simulink model "trippel_oppdatert_sim"  (R2023b)
settings: Solver=VariableStepAuto  StartTime=0.0  StopTime=inf  FixedStep=0.0001  RelTol=1e-6  AbsTol=1e-6
model workspace (MAT data in the model file):
  SL_ROS_VariableLengthArrays_MaxSizes.CommonInfo.ArrayTruncateAction = 'EmitWarning'
  SL_ROS_VariableLengthArrays_MaxSizes.MsgTypeMap = containers.Map
  SL_ROS_VariableLengthArrays_MaxSizes.MsgTypeMap.serialization.keys = {'std_msgs/Float64MultiArray'}
  SL_ROS_VariableLengthArrays_MaxSizes.MsgTypeMap.serialization.values{1}.PropertyName = 'data'
  SL_ROS_VariableLengthArrays_MaxSizes.MsgTypeMap.serialization.values{1}.DataType = 'double'
  SL_ROS_VariableLengthArrays_MaxSizes.MsgTypeMap.serialization.values{1}.MaxLength = 500
  SL_ROS_VariableLengthArrays_MaxSizes.MsgTypeMap.serialization.uniformity = 0
  SL_ROS_VariableLengthArrays_MaxSizes.MsgTypeMap.serialization.keyType = 'char'
  SL_ROS_VariableLengthArrays_MaxSizes.MsgTypeMap.serialization.valueType = 'any'
values from neighbouring files (symbols this model uses):
  Iz = (1/12) * m * (with^2 + len^2)    [LoneWolfParams.m]
  m = 375    [LoneWolfParams.m]
  wheelRadius = 0.33    [LoneWolfParams.m]
  xdotinit = 1e-3    (= 0.001)    [LoneWolfParams.m]
undefined symbols (not defined in the file or in its folder): alpha_peak, Bc, Bl, Cc, Cl, Dc, Dl, Ec, El, kappa_peak, latitude, longitude
libraries: ros2lib x11, sldrtlib x1
settings Model: Creator=bakke  LastModifiedBy=lonewolf
settings SolverCC: AutoScaleAbsTol=off  EnableFixedStepZeroCrossing=on  MaxZcBracketingIterations=100
settings OptimizationCC: EnhancedBackFolding=on  PassReuseOutputArgsAs=Individual arguments  ZeroExternalMemoryAtStartup=off  ZeroInternalMemoryAtStartup=off  MaxStackSize=64  OptimizeBlockOrder=speed  DifferentSizesBufferReuse=on  EfficientTunableParamExpr=on
settings DebuggingCC: ParameterTunabilityLossMsg=error
settings HardwareCC: ProdBitPerLong=64  ProdHWDeviceType=Intel->x86-64 (Linux 64)  UseEmbeddedCoderFeatures=off
settings RTWCC: Description=Embedded Coder  SystemTargetFile=ert.tlc  HardwareBoard=Robot Operating System 2 (ROS 2)  TLCOptions="-aInlineSetEventsForThisBaseRateFcn=TLC_FALSE -aSuppressMultiTaskScheduler=TLC_FALSE  -aRateBasedStepFcn=0"  TemplateMakefile=ert_default_tmf  Toolchain=Colcon Tools  TargetLang=C++
settings CodeAppCC: ForceParamTrailComments=on  IgnoreCustomStorageClasses=off  OperatorAnnotations=on  SimulinkDataObjDesc=on  SFDataObjDesc=on  InsertBlockDesc=on
settings ERTTargetCC: CodeInterfacePackaging=C++ class  SupportNonInlinedSFcns=on  RootIOFormat=Structure reference

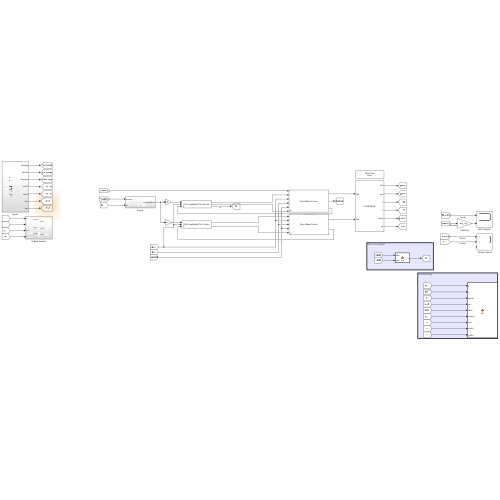
[thumbnail: Simulink's stored preview of the top-level diagram]
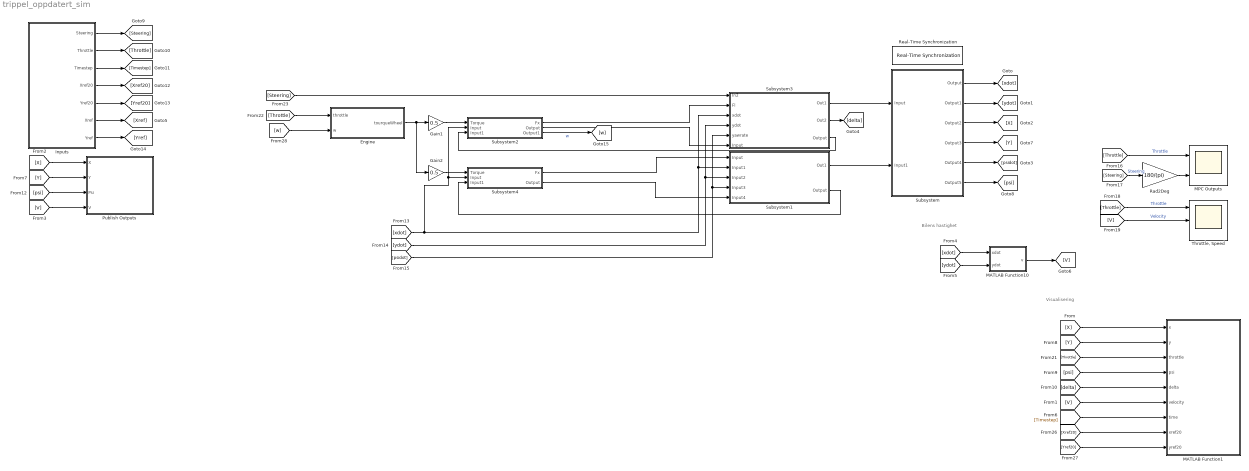
== system trippel_oppdatert_sim ==
  note: Visualisering
  note: Bilens hastighet
  Engine : Subsystem
  Gain1 : Gain  Gain=0.5
  Gain2 : Gain  Gain=0.5
  Inputs : Subsystem
  MATLAB Function1 : MATLAB Function  TreatAsAtomicUnit=on
  MATLAB Function10 : MATLAB Function  TreatAsAtomicUnit=on
  MPC Outputs : Scope  NumInputPorts=2
  Publish Outputs : Subsystem
  Rad2Deg : Gain  Gain=180/(pi)
  Real-Time Synchronization : sldrtlib/Real-Time Synchronization  SampleTime=0.1  MaxMissedTicks=1000  ShowMissedTicks=off  YieldWhenWaiting=off
  Subsystem : Subsystem
      mask Display: disp('LONE WOLF');
  Subsystem1 : Subsystem
      mask Display: disp('Rear Wheel Forces');
  Subsystem2 : Subsystem
      mask Display: disp('FW Longitudinal Tire Forces');
  Subsystem3 : Subsystem
      mask Display: disp('Front Wheel Forces');
  Subsystem4 : Subsystem
      mask Display: disp('RW Longitudinal Tire Forces');
  "Throttle, Speed" : Scope  NumInputPorts=3
  wires:
  MATLAB Function10/1(v) -> [V]
  [ydot] -> MATLAB Function10/2(ydot)
  Subsystem/1(Output) -> [xdot]
  [xdot] -> MATLAB Function10/1(xdot)
  Subsystem/2(Output1) -> [ydot]
  Subsystem/5(Output4) -> [psidot]
  Subsystem/4(Output3) -> [Y]
  Subsystem/3(Output2) -> [X]
  Subsystem/6(Output5) -> [psi]
  Subsystem1/1(Out1) -> Subsystem/2(Input1)
  Subsystem3/1(Out1) -> Subsystem/1(Input)
  [xdot] -> Subsystem4/2(Input), Subsystem2/2(Input), Subsystem3/3(xdot), Subsystem1/2(Input1)
  [ydot] -> Subsystem1/3(Input2), Subsystem3/4(ydot)
  [psidot] -> Subsystem3/5(yawrate), Subsystem1/4(Input3)
  Subsystem3/2(Out2) -> [delta]
  [X] -> MATLAB Function1/1(x)
  [Y] -> MATLAB Function1/2(y)
  [psi] -> MATLAB Function1/4(psi)
  [delta] -> MATLAB Function1/5(delta)
  [X] -> Publish Outputs/1(X)
  [Y] -> Publish Outputs/2(Y)
  [psi] -> Publish Outputs/3(Psi)
  [V] -> Publish Outputs/4(V)
  [V] -> MATLAB Function1/6(velocity)
  Inputs/1(Steering) -> [Steering]
  Inputs/2(Throttle) -> [Throttle]
  [Throttle] -> MPC Outputs/1  "Throttle"
  [Steering] -> Rad2Deg/1  "Steering"
  [Throttle] -> "Throttle, Speed"/1  "Throttle"
  [V] -> "Throttle, Speed"/2  "Velocity"
  Rad2Deg/1 -> MPC Outputs/2
  Inputs/3(Timestep) -> [Timestep]
  Inputs/4(Xref20) -> [Xref20]
  Inputs/5(Yref20) -> [Yref20]
  Subsystem2/1(Fx) -> Subsystem3/2(Fl)
  Gain1/1 -> Subsystem2/1(Torque)
  Engine/1(tourqueWheel) -> Gain2/1, Gain1/1
  Gain2/1 -> Subsystem4/1(Torque)
  Subsystem2/2(Output) -> Subsystem3/6(Input)
  Subsystem4/1(Fx) -> Subsystem1/1(Input)
  Subsystem4/2(Output) -> Subsystem1/5(Input4)
  Inputs/6(Xref) -> [Xref]
  Inputs/7(Yref) -> [Yref]
  Subsystem2/3(Output1) -> [w]  "w"
  [Steering] -> Subsystem3/1(In2)
  [w] -> Engine/2(w)
  Subsystem1/2(Output) -> Subsystem4/3(Input1)
  Subsystem3/3(Output) -> Subsystem2/3(Input1)
  [Yref20] -> MATLAB Function1/9(yref20)
  [Xref20] -> MATLAB Function1/8(xref20)
  [Throttle] -> MATLAB Function1/3(throttle)
  [Timestep] -> MATLAB Function1/7(time)
  [Throttle] -> Engine/1(throttle)

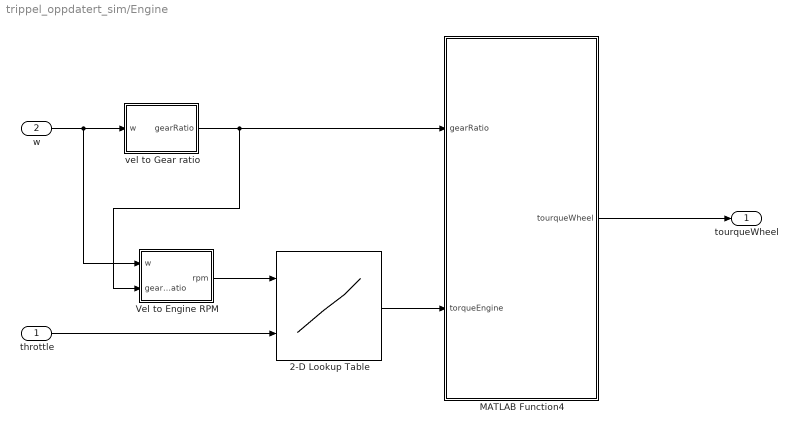
== system trippel_oppdatert_sim/Engine ==
  throttle : Inport
  w : Inport  Port=2
  2-D Lookup Table : Lookup_n-D  BreakpointsForDimension1=[0;169.614855264094;367.085957899886;589.246670617181;789.821522752712;996.567251474744;1181.71186027627;1425.48895225281;1626.06685625609;1835.92854194885;2042.68342627413;2243.26743401291;2425.36017506641;2616.68481605769;2860.48021924071;3085.77825200297;3264.76724355674;3468.45194892751;3656.70641096427;3909.77338836579;4131.97377536381;4314.05736081407;4493.04635236784;4696.71885026762;4909.65376678264;5110.24998199241;5292.32135997168;5499.07014056146;5718.17288179523;5965.03541206502;6199.56534476505;6390.87472641759;6582.16884873138;6758.05409078541;6980.20259603171]  BreakpointsForDimension2=[0;10;20;30;40;50;60;70;80;90;100]  Table=[0.3 7.52683562951347 11.8387627553835 13.7538912505429 14.2370681748395 17.110514311951 18.5474885119643 17.5896731329271 18.0683296909882 19.0271495958556 24.298398889508;0.2 10.3686392029757 12.7749808290727 17.5615464096832 19.4852133743988 21.8820120051095 25.2300965969615 24.7539513534759 28.0985201049223 31.4546409034155 33.8484259566359;0 11.2978255958539 15.1431504736246 22.3255101591157 25.2084992916136 29.038254019017 37.6505562237105 34.7881598707304 46.2688855833847 47.2272032253369 51.5386280882919;0 13.1858318935994 20.8624182875188 30.4380607633152 37.1492978344714 39.5491100426724 54.8631063231358 53.915838465315 65.4061071733557 67.8013990153211 73.0706392573133;0 16.0346671478725 30.4094317771563 43.3462176805965 52.4527465937181 63.4723949503387 69.6994505713682 77.3680007586463 84.553876284543 88.8678124620733 88.8688169879034;-2.44629412790408 24.6344127796893 47.1563841543122 73.0294536982776 73.0379921678338 91.720665819667 102.743327753778 118.552053005585 116.160277004025 127.660088707451 124.308990538109;-4.96800884998436 35.1502914324955 71.0816781136389 103.177785175313 114.222546677687 132.430079611865 148.722986313798 180.336920977006 188.48362545943 193.279734035427 163.107293938468;-8.74578514092923 33.6856927721534 72.4880142758329 104.587637177913 130.961462848202 155.87470796147 177.437859431226 195.635347107102 209.529446126664 221.029760093006 226.319090851601;-12.1015317204333 33.6520411568438 75.3288133234649 113.858360154898 143.370370427905 164.462399283325 190.810609544946 214.287382721116 229.13779033097 243.993220569975 247.83502960734;-19.201920026761 35.0558660044625 81.0551128181702 121.980453754484 158.198176206581 185.034586021649 211.865973207567 232.947956804686 250.676330917887 265.053104598831 277.032075123234;-23.3903905203684 35.0282415441337 84.3810978417591 127.227594428213 165.359943112554 196.510289105152 225.735461344291 249.691393341436 267.899930801444 284.190326188802 296.649460060012;-27.5779890517621 31.4144554912304 86.2680996136746 133.424012011423 173.479023134649 206.067347853091 234.811352219593 263.073686450543 283.200365983201 296.143179041622 314.343680294988;-34.6744535281279 28.5083622646395 84.8029986904173 132.424508810435 174.403689161292 210.348636941142 239.083600575173 265.9119741836 288.438465924458 303.782095716911 318.144303773318;-38.4448181402563 22.7303296896822 79.0219525379695 127.60881198075 170.065644363838 207.922707061357 236.655159380812 261.571418071571 285.059241031872 302.791633248394 315.243735438792;-44.7181502868699 19.3501002712657 76.5965249210998 125.188909255946 170.034504063104 205.489745500762 237.114227685186 262.989306280812 284.552457750567 303.239651768636 317.613914135005;-53.0684964265662 14.5328966528359 72.7336208413018 123.725817384349 168.093257896361 204.501292083905 235.646615447353 263.444356481864 285.961807490252 304.168335898599 318.061932655246;-57.6689690661566 10.1943495924673 67.9169194857871 119.863917830381 165.197712190987 201.122569454234 232.254331718975 261.012399447099 284.010516065207 301.740396967154 318.513467015894;-63.9366334583809 4.41481022876471 62.1353710704242 114.762859997277 162.775298151607 195.485378400082 228.870586460153 255.707498538137 277.747799777208 296.440518687343 312.256777882875;-69.7861919691262 -2.32304677689018 58.7496167599421 109.939629223867 157.474917608881 193.058946257382 225.968009073968 255.203226571407 278.19581829745 296.410885175354 312.707307717692;-78.1404619387842 -9.54508523267177 53.452249794706 105.592543693942 154.556770072328 190.157373397027 224.031785536375 252.782821583688 275.782444990542 295.429463439308 311.718854300836;-84.8266681935945 -12.4471603559423 48.6390642795968 102.692979885247 151.179554231402 188.687752107534 223.0493592745 251.318725186261 274.317344067285 293.481687854669 309.292422158136;-90.6753547421262 -16.3085576469951 45.7379936821564 99.7888957103159 147.799324812986 188.655607280969 222.54508730777 250.807923801635 ...(+2434 chars)]  InternalRulePriority=Speed  RndMeth=Simplest
      settings: InputPortMap=u0,u1
  MATLAB Function4 : MATLAB Function  TreatAsAtomicUnit=on
  Vel to Engine RPM : MATLAB Function  TreatAsAtomicUnit=on
  vel to Gear ratio : MATLAB Function  TreatAsAtomicUnit=on
  tourqueWheel : Outport
  wires:
  vel to Gear ratio/1(gearRatio) -> Vel to Engine RPM/2(gearRatio), MATLAB Function4/1(gearRatio)
  2-D Lookup Table/1 -> MATLAB Function4/2(torqueEngine)
  MATLAB Function4/1(tourqueWheel) -> tourqueWheel/1
  throttle/1 -> 2-D Lookup Table/2
  w/1 -> vel to Gear ratio/1(w), Vel to Engine RPM/1(w)
  Vel to Engine RPM/1(rpm) -> 2-D Lookup Table/1

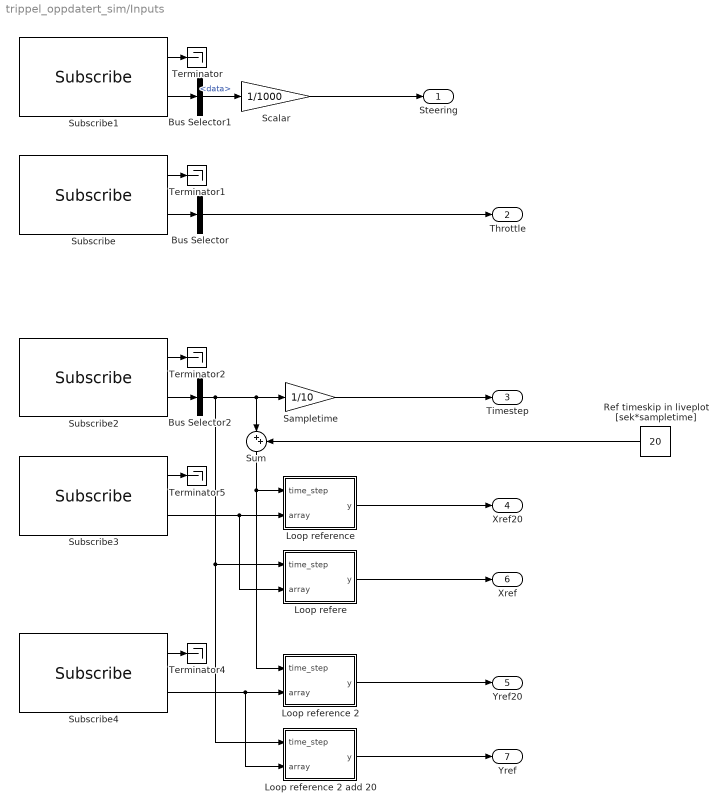
== system trippel_oppdatert_sim/Inputs ==
  Bus Selector : BusSelector  OutputSignals=data  OutputAsBus=on
  Bus Selector1 : BusSelector  OutputSignals=data
  Bus Selector2 : BusSelector  OutputSignals=data  OutputAsBus=on
  Loop refere : MATLAB Function  TreatAsAtomicUnit=on
  Loop reference : MATLAB Function  TreatAsAtomicUnit=on
  Loop reference 2 : MATLAB Function  TreatAsAtomicUnit=on
  Loop reference 2 add 20 : MATLAB Function  TreatAsAtomicUnit=on
  Ref timeskip in liveplot [sek*sampletime] : Constant  Value=20
  Sampletime : Gain  Gain=1/10
  Scalar : Gain  Gain=1/1000
  Subscribe : ros2lib/Subscribe  topicSource=Specify your own  topic=/lw_portenta_throttle  messageType=std_msgs/Int64  sampleTime=0.1  QOSHistory=Keep last  QOSDepth=1  QOSReliability=Reliable  QOSDurability=Volatile
  Subscribe1 : ros2lib/Subscribe  topicSource=Specify your own  topic=/lw_portenta_steering  messageType=std_msgs/Int64  sampleTime=0.1  QOSHistory=Keep last  QOSDepth=1  QOSReliability=Reliable  QOSDurability=Volatile
  Subscribe2 : ros2lib/Subscribe  topicSource=Specify your own  topic=/timestep  messageType=std_msgs/Int64  sampleTime=0.1  QOSHistory=Keep last  QOSDepth=1  QOSReliability=Reliable  QOSDurability=Volatile
  Subscribe3 : ros2lib/Subscribe  topicSource=Specify your own  topic=/xref  messageType=std_msgs/Float64MultiArray  sampleTime=0.1  QOSHistory=Keep last  QOSDepth=1  QOSReliability=Reliable  QOSDurability=Volatile
  Subscribe4 : ros2lib/Subscribe  topicSource=Specify your own  topic=/yref  messageType=std_msgs/Float64MultiArray  sampleTime=0.1  QOSHistory=Keep last  QOSDepth=1  QOSReliability=Reliable  QOSDurability=Volatile
  Sum : Sum  Inputs=|++
  Terminator{,1..2,4..5} (5 alike) : Terminator
  Steering : Outport
  Throttle : Outport  Port=2
  Timestep : Outport  Port=3
  Xref20 : Outport  Port=4
  Yref20 : Outport  Port=5
  Xref : Outport  Port=6
  Yref : Outport  Port=7
  wires:
  Subscribe/1 -> Terminator1/1
  Subscribe1/1 -> Terminator/1
  Subscribe/2 -> Bus Selector/1
  Subscribe1/2 -> Bus Selector1/1
  Bus Selector1/1 -> Scalar/1  "<data>"
  Bus Selector/1 -> Throttle/1
  Scalar/1 -> Steering/1
  Subscribe2/1 -> Terminator2/1
  Subscribe2/2 -> Bus Selector2/1
  Bus Selector2/1 -> Loop refere/1(time_step), Loop reference 2 add 20/1(time_step), Sum/1, Sampletime/1
  Sampletime/1 -> Timestep/1
  Subscribe4/1 -> Terminator4/1
  Subscribe4/2 -> Loop reference 2 add 20/2(array), Loop reference 2/2(array)
  Subscribe3/2 -> Loop refere/2(array), Loop reference/2(array)
  Subscribe3/1 -> Terminator5/1
  Ref timeskip in liveplot [sek*sampletime]/1 -> Sum/2
  Sum/1 -> Loop reference/1(time_step), Loop reference 2/1(time_step)
  Loop reference/1(y) -> Xref20/1
  Loop refere/1(y) -> Xref/1
  Loop reference 2 add 20/1(y) -> Yref/1
  Loop reference 2/1(y) -> Yref20/1

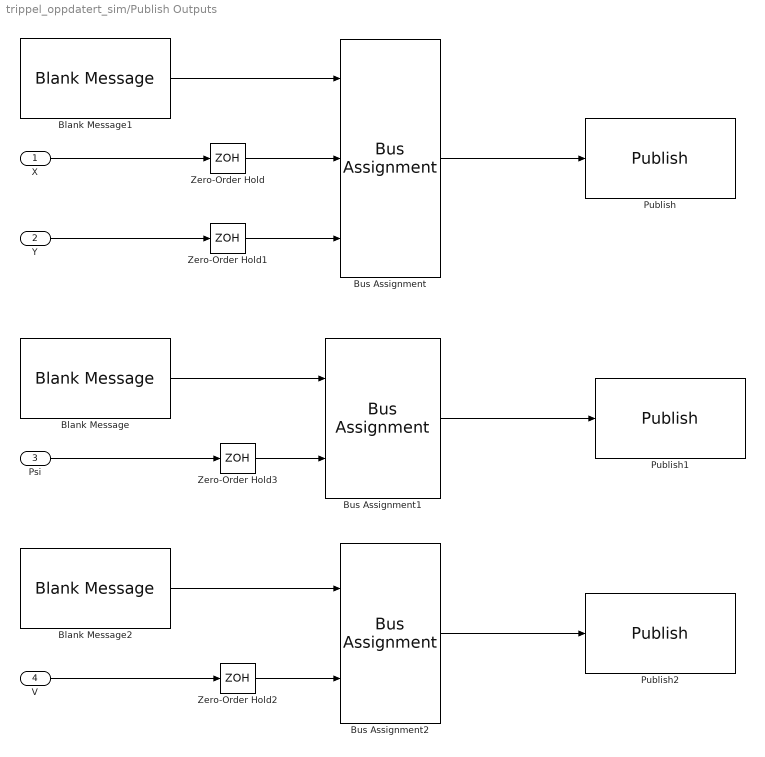
== system trippel_oppdatert_sim/Publish Outputs ==
  X : Inport
  Y : Inport  Port=2
  Psi : Inport  Port=3
  V : Inport  Port=4
  Blank Message : ros2lib/Blank Message  messageClass=Message  entityType=geometry_msgs/PoseWithCovarianceStamped  messageType=geometry_msgs/PoseWithCovarianceStamped  SampleTime=0.1
  Blank Message1 : ros2lib/Blank Message  messageClass=Message  entityType=sensor_msgs/NavSatFix  messageType=sensor_msgs/NavSatFix  SampleTime=0.1
  Blank Message2 : ros2lib/Blank Message  messageClass=Message  entityType=geometry_msgs/TwistWithCovarianceStamped  messageType=geometry_msgs/TwistWithCovarianceStamped  SampleTime=0.1
  Bus Assignment : BusAssignment  AssignedSignals=latitude,longitude
  Bus Assignment1 : BusAssignment  AssignedSignals=pose.pose.position.z
  Bus Assignment2 : BusAssignment  AssignedSignals=twist.twist.linear.x
  Publish : ros2lib/Publish  topicSource=Specify your own  topic=/vectornav/gnss  messageType=sensor_msgs/NavSatFix  QOSHistory=Keep last  QOSDepth=1  QOSReliability=Reliable  QOSDurability=Volatile
  Publish1 : ros2lib/Publish  topicSource=Specify your own  topic=/vectornav/pose  messageType=geometry_msgs/PoseWithCovarianceStamped  QOSHistory=Keep last  QOSDepth=1  QOSReliability=Reliable  QOSDurability=Volatile
  Publish2 : ros2lib/Publish  topicSource=Specify your own  topic=/vectornav/velocity_body  messageType=geometry_msgs/TwistWithCovarianceStamped  QOSHistory=Keep last  QOSDepth=1  QOSReliability=Reliable  QOSDurability=Volatile
  Zero-Order Hold{,1..3} (4 alike) : ZeroOrderHold  SampleTime=0.1
  wires:
  Blank Message/1 -> Bus Assignment1/1
  Bus Assignment1/1 -> Publish1/1
  Zero-Order Hold2/1 -> Bus Assignment2/2
  Bus Assignment2/1 -> Publish2/1
  Zero-Order Hold3/1 -> Bus Assignment1/2
  Psi/1 -> Zero-Order Hold3/1
  Blank Message1/1 -> Bus Assignment/1
  V/1 -> Zero-Order Hold2/1
  X/1 -> Zero-Order Hold/1
  Zero-Order Hold/1 -> Bus Assignment/2
  Bus Assignment/1 -> Publish/1
  Blank Message2/1 -> Bus Assignment2/1
  Y/1 -> Zero-Order Hold1/1
  Zero-Order Hold1/1 -> Bus Assignment/3

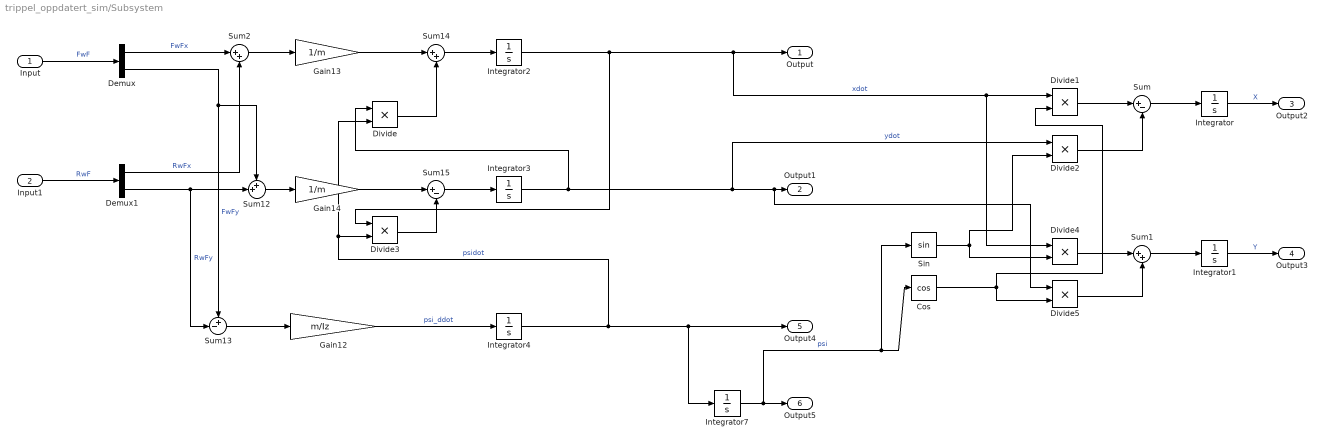
== system trippel_oppdatert_sim/Subsystem ==
  Input : Inport
  Input1 : Inport  Port=2
  Cos : Trigonometry  Operator=cos
  Demux : Demux  Outputs=2
  Demux1 : Demux  Outputs=2
  Divide{,1..5} (6 alike) : Product  Inputs=**
  Gain12 : Gain  Gain=m/Iz
  Gain13 : Gain  Gain=1/m
  Gain14 : Gain  Gain=1/m
  Integrator{,1,3..4,7} (5 alike) : Integrator
  Integrator2 : Integrator  InitialCondition=xdotinit
  Sin : Trigonometry
  Sum : Sum  Inputs=|+-
  Sum1 : Sum  Inputs=|++
  Sum12 : Sum  Inputs=++|
  Sum13 : Sum  Inputs=+-|
  Sum14 : Sum  Inputs=|++
  Sum15 : Sum  Inputs=|+-
  Sum2 : Sum  Inputs=|++
  Output : Outport
  Output1 : Outport  Port=2
  Output2 : Outport  Port=3
  Output3 : Outport  Port=4
  Output4 : Outport  Port=5
  Output5 : Outport  Port=6
  wires:
  Demux1/1 -> Sum2/2  "RwFx"
  Input/1 -> Demux/1  "FwF"
  Demux/1 -> Sum2/1  "FwFx"
  Demux1/2 -> Sum12/2, Sum13/2  "RwFy"
  Integrator2/1 -> Divide1/1, Divide4/1, Output/1, Divide3/1  "xdot"
  Sum13/1 -> Gain12/1
  Integrator4/1 -> Output4/1, Integrator7/1, Divide3/2, Divide/2  "psidot"
  Sum14/1 -> Integrator2/1
  Demux/2 -> Sum12/1, Sum13/1  "FwFy"
  Input1/1 -> Demux1/1  "RwF"
  Gain13/1 -> Sum14/1
  Integrator7/1 -> Output5/1, Cos/1, Sin/1  "psi"
  Gain14/1 -> Sum15/1
  Integrator3/1 -> Divide5/1, Output1/1, Divide2/1, Divide/1  "ydot"
  Divide3/1 -> Sum15/2
  Gain12/1 -> Integrator4/1  "psi_ddot"
  Sum2/1 -> Gain13/1
  Sum15/1 -> Integrator3/1
  Sum12/1 -> Gain14/1
  Divide/1 -> Sum14/2
  Cos/1 -> Divide5/2, Divide1/2
  Sin/1 -> Divide4/2, Divide2/2
  Divide1/1 -> Sum/1
  Divide2/1 -> Sum/2
  Divide4/1 -> Sum1/1
  Divide5/1 -> Sum1/2
  Sum/1 -> Integrator/1
  Integrator/1 -> Output2/1  "X"
  Sum1/1 -> Integrator1/1
  Integrator1/1 -> Output3/1  "Y"

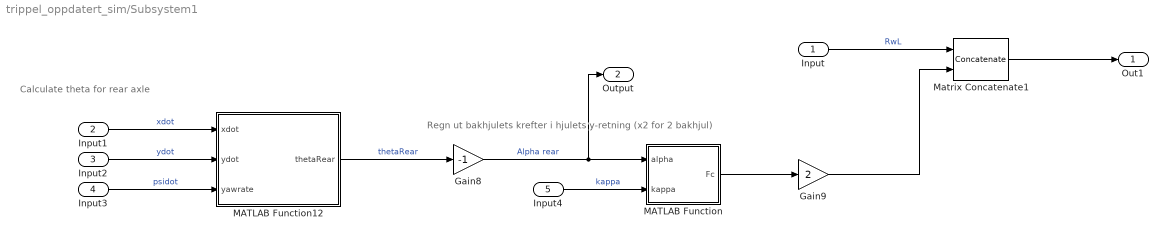
== system trippel_oppdatert_sim/Subsystem1 ==
  note: Regn ut bakhjulets krefter i hjulets y-retning (x2 for 2 bakhjul)
  note: Calculate theta for rear axle
  Input : Inport
  Input1 : Inport  Port=2
  Input2 : Inport  Port=3
  Input3 : Inport  Port=4
  Input4 : Inport  Port=5
  Gain8 : Gain  Gain=-1
  Gain9 : Gain  Gain=2
  MATLAB Function : MATLAB Function  TreatAsAtomicUnit=on
  MATLAB Function12 : MATLAB Function  TreatAsAtomicUnit=on
  Matrix Concatenate1 : Concatenate  Mode=Multidimensional array
  Out1 : Outport
  Output : Outport  Port=2
  wires:
  Matrix Concatenate1/1 -> Out1/1
  Gain8/1 -> MATLAB Function/1(alpha), Output/1  "Alpha rear"
  MATLAB Function12/1(thetaRear) -> Gain8/1  "thetaRear"
  Gain9/1 -> Matrix Concatenate1/2
  Input/1 -> Matrix Concatenate1/1  "RwL"
  Input3/1 -> MATLAB Function12/3(yawrate)  "psidot"
  Input2/1 -> MATLAB Function12/2(ydot)  "ydot"
  Input1/1 -> MATLAB Function12/1(xdot)  "xdot"
  MATLAB Function/1(Fc) -> Gain9/1
  Input4/1 -> MATLAB Function/2(kappa)  "kappa"

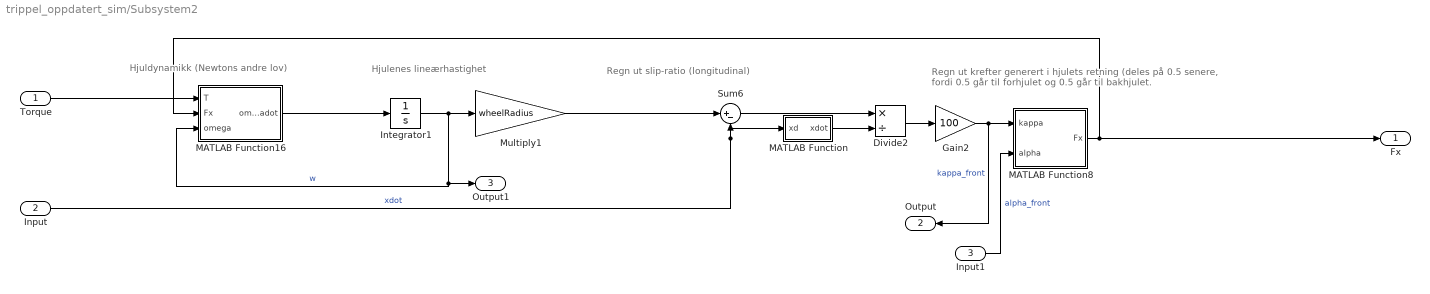
== system trippel_oppdatert_sim/Subsystem2 ==
  note: Hjulenes lineærhastighet
  note: Regn ut krefter generert i hjulets retning (deles på 0.5 senere, fordi 0.5 går til forhjulet og 0.5 går til bakhjulet.
  note: Regn ut slip-ratio (longitudinal)
  note: Hjuldynamikk (Newtons andre lov)
  Torque : Inport
  Input : Inport  Port=2
  Input1 : Inport  Port=3
  Divide2 : Product  Inputs=*/
  Gain2 : Gain  Gain=100
  Integrator1 : Integrator  InitialCondition=(xdotinit)/0.3
  MATLAB Function : MATLAB Function  TreatAsAtomicUnit=on
  MATLAB Function16 : MATLAB Function  TreatAsAtomicUnit=on
  MATLAB Function8 : MATLAB Function  TreatAsAtomicUnit=on
  Multiply1 : Gain  Gain=wheelRadius
  Sum6 : Sum  Inputs=|+-
  Fx : Outport
  Output : Outport  Port=2
  Output1 : Outport  Port=3
  wires:
  MATLAB Function8/1(Fx) -> Fx/1, MATLAB Function16/2(Fx)
  Divide2/1 -> Gain2/1
  MATLAB Function16/1(omegadot) -> Integrator1/1
  Integrator1/1 -> Multiply1/1, Output1/1, MATLAB Function16/3(omega)  "w"
  Multiply1/1 -> Sum6/1
  Sum6/1 -> Divide2/1
  Input/1 -> MATLAB Function/1(xd), Sum6/2  "xdot"
  MATLAB Function/1(xdot) -> Divide2/2
  Gain2/1 -> MATLAB Function8/1(kappa), Output/1  "kappa_front"
  Torque/1 -> MATLAB Function16/1(T)
  Input1/1 -> MATLAB Function8/2(alpha)  "alpha_front"

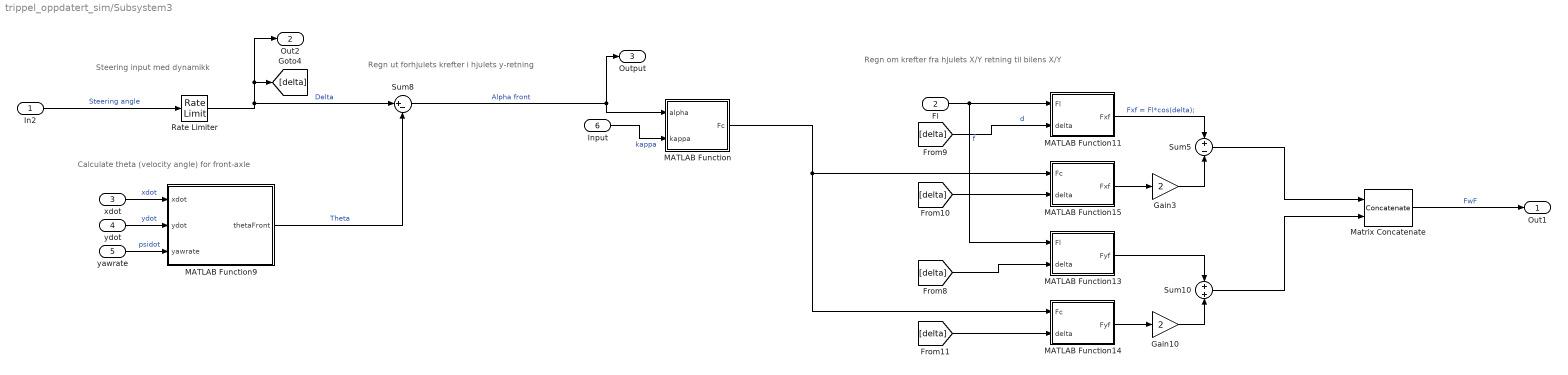
== system trippel_oppdatert_sim/Subsystem3 ==
  note: Regn om krefter fra hjulets X/Y retning til bilens X/Y
  note: Steering input med dynamikk
  note: Regn ut forhjulets krefter i hjulets y-retning
  note: Calculate theta (velocity angle) for front-axle
  In2 : Inport
  Fl : Inport  Port=2
  xdot : Inport  Port=3
  ydot : Inport  Port=4
  yawrate : Inport  Port=5
  Input : Inport  Port=6
  Gain10 : Gain  Gain=2
  Gain3 : Gain  Gain=2
  MATLAB Function : MATLAB Function  TreatAsAtomicUnit=on
  MATLAB Function11 : MATLAB Function  TreatAsAtomicUnit=on
  MATLAB Function13 : MATLAB Function  TreatAsAtomicUnit=on
  MATLAB Function14 : MATLAB Function  TreatAsAtomicUnit=on
  MATLAB Function15 : MATLAB Function  TreatAsAtomicUnit=on
  MATLAB Function9 : MATLAB Function  TreatAsAtomicUnit=on
  Matrix Concatenate : Concatenate  Mode=Multidimensional array
  Rate Limiter : RateLimiter  RisingSlewLimit=pi/2  FallingSlewLimit=-pi/2
  Sum10 : Sum  Inputs=+|+
  Sum5 : Sum  Inputs=+|-
  Sum8 : Sum  Inputs=|+-
  Out1 : Outport
  Out2 : Outport  Port=2
  Output : Outport  Port=3
  wires:
  Gain3/1 -> Sum5/2
  Sum10/1 -> Matrix Concatenate/2
  MATLAB Function11/1(Fxf) -> Sum5/1  "Fxf = Fl*cos(delta);"
  [delta] -> MATLAB Function11/2(delta)  "d"
  MATLAB Function15/1(Fxf) -> Gain3/1
  Sum5/1 -> Matrix Concatenate/1
  [delta] -> MATLAB Function15/2(delta)
  MATLAB Function9/1(thetaFront) -> Sum8/2  "Theta"
  Gain10/1 -> Sum10/2
  [delta] -> MATLAB Function14/2(delta)
  MATLAB Function13/1(Fyf) -> Sum10/1
  Sum8/1 -> Output/1, MATLAB Function/1(alpha)  "Alpha front"
  MATLAB Function14/1(Fyf) -> Gain10/1
  [delta] -> MATLAB Function13/2(delta)
  Rate Limiter/1 -> [delta], Out2/1, Sum8/1  "Delta"
  Matrix Concatenate/1 -> Out1/1  "FwF"
  In2/1 -> Rate Limiter/1  "Steering angle"
  Fl/1 -> MATLAB Function11/1(Fl), MATLAB Function13/1(Fl)  "f"
  xdot/1 -> MATLAB Function9/1(xdot)  "xdot"
  ydot/1 -> MATLAB Function9/2(ydot)  "ydot"
  yawrate/1 -> MATLAB Function9/3(yawrate)  "psidot"
  MATLAB Function/1(Fc) -> MATLAB Function15/1(Fc), MATLAB Function14/1(Fc)
  Input/1 -> MATLAB Function/2(kappa)  "kappa"

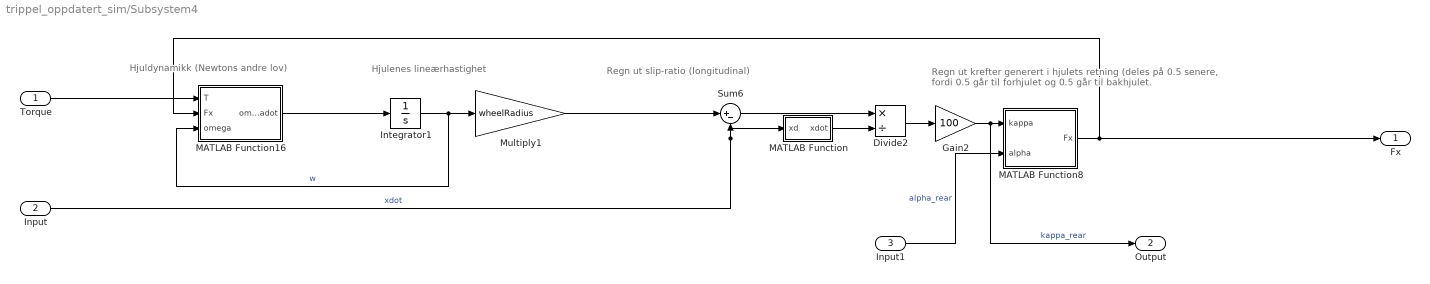
== system trippel_oppdatert_sim/Subsystem4 ==
  note: Hjulenes lineærhastighet
  note: Regn ut krefter generert i hjulets retning (deles på 0.5 senere, fordi 0.5 går til forhjulet og 0.5 går til bakhjulet.
  note: Regn ut slip-ratio (longitudinal)
  note: Hjuldynamikk (Newtons andre lov)
  Torque : Inport
  Input : Inport  Port=2
  Input1 : Inport  Port=3
  Divide2 : Product  Inputs=*/
  Gain2 : Gain  Gain=100
  Integrator1 : Integrator  InitialCondition=(xdotinit)/0.3
  MATLAB Function : MATLAB Function  TreatAsAtomicUnit=on
  MATLAB Function16 : MATLAB Function  TreatAsAtomicUnit=on
  MATLAB Function8 : MATLAB Function  TreatAsAtomicUnit=on
  Multiply1 : Gain  Gain=wheelRadius
  Sum6 : Sum  Inputs=|+-
  Fx : Outport
  Output : Outport  Port=2
  wires:
  MATLAB Function8/1(Fx) -> Fx/1, MATLAB Function16/2(Fx)
  Divide2/1 -> Gain2/1
  MATLAB Function16/1(omegadot) -> Integrator1/1
  Integrator1/1 -> Multiply1/1, MATLAB Function16/3(omega)  "w"
  Multiply1/1 -> Sum6/1
  Sum6/1 -> Divide2/1
  Input/1 -> MATLAB Function/1(xd), Sum6/2  "xdot"
  MATLAB Function/1(xdot) -> Divide2/2
  Gain2/1 -> MATLAB Function8/1(kappa), Output/1  "kappa_rear"
  Torque/1 -> MATLAB Function16/1(T)
  Input1/1 -> MATLAB Function8/2(alpha)  "alpha_rear"

== matlab function trippel_oppdatert_sim/Subsystem4/MATLAB Function16 ==
  data: T input; omegadot output; Fx input; omega input
function omegadot = fcn(T, Fx, omega)

omegadot = (T - 0.33 * Fx - 5 * omega)/0.5;

% 0.5 = Hjulets treghetsmoment
% 8 * omega motorbrems / rullemotstand

== matlab function trippel_oppdatert_sim/Subsystem2/MATLAB Function8 ==
  data: Fx output; Bl parameter; Cl parameter; Dl parameter; El parameter; kappa_peak parameter; alpha_peak parameter; kappa input; alpha input
function Fx = fcn(Bl, Cl, Dl, El, kappa_peak, alpha_peak, kappa, alpha)

alpha_norm = alpha/alpha_peak;
kappa_norm = kappa/kappa_peak;

S = sqrt(alpha_norm^2+kappa_norm^2);

kappa_mod = S * alpha_peak;

Fx = kappa_norm/S * Dl*sin(Cl*atan(Bl*kappa_mod-El*(Bl*kappa_mod-atan(Bl*kappa_mod))));

== matlab function trippel_oppdatert_sim/Subsystem3/MATLAB Function9 ==
  data: xdot input; thetaFront output; ydot input; yawrate input
function thetaFront = fcn(xdot, ydot, yawrate)

thetaFront = atan((ydot+yawrate*1.4)/xdot);

== matlab function trippel_oppdatert_sim/Subsystem1/MATLAB Function12 ==
  data: xdot input; thetaRear output; ydot input; yawrate input
function thetaRear = fcn(xdot, ydot, yawrate)

thetaRear = atan((ydot-yawrate*1.6)/xdot);

== matlab function trippel_oppdatert_sim/Subsystem3/MATLAB Function13 ==
  data: Fl input; Fyf output; delta input
function Fyf = fcn(Fl, delta)

Fyf = Fl*sin(delta);

== matlab function trippel_oppdatert_sim/Subsystem3/MATLAB Function14 ==
  data: Fc input; delta input; Fyf output
function Fyf = fcn(Fc, delta)

Fyf = Fc*cos(delta);

== matlab function trippel_oppdatert_sim/Subsystem3/MATLAB Function15 ==
  data: Fc input; Fxf output; delta input
function Fxf = fcn(Fc, delta)

Fxf = Fc*sin(delta);

== matlab function trippel_oppdatert_sim/Subsystem2/MATLAB Function16 ==
  data: T input; omegadot output; Fx input; omega input
function omegadot = fcn(T, Fx, omega)

omegadot = (T - 0.33 * Fx - 5 * omega)/0.5;

% 0.5 = Hjulets treghetsmoment
% 8 * omega motorbrems / rullemotstand

== matlab function trippel_oppdatert_sim/Engine/Vel to Engine RPM ==
  data: w input; rpm output; gearRatio input
function rpm = fcn(w,gearRatio)


rpm = (w*9.55)*gearRatio*4.04;

== matlab function trippel_oppdatert_sim/Engine/vel to Gear ratio ==
  data: w input; gearRatio output
function gearRatio = fcn(w)

velLimitLow = 3.72;
velLimitHigh = 12;
lowRatio = 5.952;
highRatio = 3.691;
velocity = w*0.33;

if (velocity < velLimitLow)
    gearRatio = lowRatio;
elseif (velLimitLow < velocity && velocity < velLimitHigh)
    gearRatio = lowRatio - (velocity-velLimitLow)/(velLimitHigh-velLimitLow)*2.26;
else
    gearRatio = highRatio;
end

== matlab function trippel_oppdatert_sim/Engine/MATLAB Function4 ==
  data: gearRatio input; torqueEngine input; tourqueWheel output
function tourqueWheel = fcn(gearRatio,torqueEngine)

tourqueWheel = torqueEngine*gearRatio* (1/2.1); % magic number shhhh scaling for 60km/h topspeed

== matlab function trippel_oppdatert_sim/Inputs/Loop refere ==
  data: time_step input; array input; y output
function y = fcn(time_step, array)
    % index = mod(time_step, N_STEPS_REFERENCE) + 1;
    index = mod(time_step, 500) + 1; 
    y = array.data(index);
end

== matlab function trippel_oppdatert_sim/Subsystem1/MATLAB Function ==
  data: alpha input; Fc output; kappa input; Bc parameter; Cc parameter; Dc parameter; Ec parameter; alpha_peak parameter; kappa_peak parameter
function Fc = fcn(alpha, kappa, Bc, Cc, Dc, Ec, alpha_peak, kappa_peak)

alpha_norm = alpha/alpha_peak;
kappa_norm = kappa/kappa_peak;

S = sqrt(alpha_norm^2+kappa_norm^2);

alpha_mod = S * alpha_peak;

Fc = alpha_norm/S * Dc*sin(Cc*atan(Bc*alpha_mod-Ec*(Bc*alpha_mod-atan(Bc*alpha_mod))));

== matlab function trippel_oppdatert_sim/MATLAB Function1 ==
  settings: updateMethod=DISCRETE  sampleTime=0.1
  data: x input; y input; throttle input; psi input; delta input; velocity input; time input; xref20 input; yref20 input
function fnc(x, y, throttle, psi, delta, velocity, time, xref20, yref20)
    persistent xmin xmax ymin ymax vehiclePathX vehiclePathY posErrorPlot errorArray refPathX refPathY vehicleFig pathPlot refPlot leftWheelPatch rightWheelPatch rearLeftWheelPatch rearRightWheelPatch lwPatch velocityPlot deltaPlot timeArray deltaArray velocityArray throttleArray throttlePlot 
    
    lwWidth = 2.4;
    lwHeight = 1.2;
    wheelWidth = 0.66;
    wheelHeight = 0.22;

    if isempty(vehicleFig)
        vehicleFig = figure('WindowState','maximized');
        hold on;
        subplot(3,6,[1:3 7:9 13:15]);
        pathPlot = plot(NaN, NaN, 'k-', 'LineWidth', 2);
        hold on;
        refPlot = plot(NaN, NaN, 'b:', 'LineWidth', 2);
        axis equal;
        grid on;
        title('Lone Wolf Simulator')
        xlabel('X-position')
        ylabel('Y-position')
        leftWheelPatch = patch('XData', [], 'YData', [], 'FaceColor', 'k', 'EdgeColor', 'k');
        rightWheelPatch = patch('XData', [], 'YData', [], 'FaceColor', 'k', 'EdgeColor', 'k');
        rearLeftWheelPatch = patch('XData', [], 'YData', [], 'FaceColor', 'k', 'EdgeColor', 'k');
        rearRightWheelPatch = patch('XData', [], 'YData', [], 'FaceColor', 'k', 'EdgeColor', 'k');
        lwPatch = patch('XData', [], 'YData', [], 'FaceColor', 'r', 'EdgeColor', 'k');
        xmin = -15;
        xmax = 15;
        ymin = -15;
        ymax = 15;

        timeArray = [];
        velocityArray = [];
        deltaArray = [];
        errorArray = [];
        throttleArray = [];

        subplot(3,6,4:6);
        velocityPlot = plot(NaN, NaN, 'g-', 'LineWidth', 2);
        hold on;
        throttlePlot = plot(NaN, NaN, 'k:', 'LineWidth', 1);
        ylabel('Velocity (km/h) | Throttle %')
        ylim([-5, 100])
        
        grid on;
        subplot(3,6,10:12);
        deltaPlot = plot(NaN, NaN, 'b-', 'LineWidth', 2);
        ylabel('Steering angle (rad)')
        ylim([-1, 1])
        grid on;
        subplot(3,6,16:18);
        posErrorPlot = plot(NaN, NaN, 'r-', 'LineWidth', 2);
        ylabel('Position error (m)')
        %ylim([-0.2, 5])
        grid on;
    end

    if isempty(refPathX)
        vehiclePathX = [];
        refPathX = [];
    end
    
    if isempty(refPathY)
        vehiclePathY = [];
        refPathY = [];
    end
    
    subplot(3,6,[1:3 7:9 13:15]);
    vehiclePathX(end+1) = x;
    vehiclePathY(end+1) = y;
    refPathX(end+1) = xref20;
    refPathY(end+1) = yref20;
    timeArray(end+1) = time;
    deltaArray(end+1) = delta;
    velocityArray(end+1) = velocity*3.6;
    throttleArray(end+1) = throttle;


    tempError = Inf;

    if length(refPathX) > 150
        t100 = 0:99;

        X100 = refPathX(end-99:end);
        Y100 = refPathY(end-99:end);
        length(t100)
        length(X100)
        length(Y100)

        tq = 0:0.002:99;
        length(tq)

        xq = interp1(t100, X100, tq, 'linear');
        yq = interp1(t100, Y100, tq, 'linear');

        for i = 1:45000
            itError = sqrt( (x - xq(end - (i)))^2 + (y - yq(end - (i)))^2 );
            if itError < tempError
                tempError = itError;
            end
        end
    end

    errorArray(end+1) = tempError;

    leftWheelVertices = [-wheelWidth/2, -wheelHeight/2;
                    wheelWidth/2, -wheelHeight/2;
                    wheelWidth/2, wheelHeight/2;
                    -wheelWidth/2, wheelHeight/2];

    rightWheelVertices = [-wheelWidth/2, -wheelHeight/2;
                    wheelWidth/2, -wheelHeight/2;
                    wheelWidth/2, wheelHeight/2;
                    -wheelWidth/2, wheelHeight/2];

    rearLeftWheelVertices = [-wheelWidth/2, -wheelHeight/2;
                    wheelWidth/2, -wheelHeight/2;
                    wheelWidth/2, wheelHeight/2;
                    -wheelWidth/2, wheelHeight/2];

    rearRightWheelVertices = [-wheelWidth/2, -wheelHeight/2;
                    wheelWidth/2, -wheelHeight/2;
                    wheelWidth/2, wheelHeight/2;
                    -wheelWidth/2, wheelHeight/2];

    lwVertices = [-lwWidth/2, -lwHeight/2;
                    lwWidth/2, -lwHeight/2;
                    lwWidth/2, lwHeight/2;
                    -lwWidth/2, lwHeight/2];
    
    R = [cos(psi), -sin(psi); sin(psi), cos(psi)];
    rotatedLW = (R * lwVertices')';
    fW = [cos(psi+delta), -sin(psi+delta); sin(psi+delta), cos(psi+delta)];
    rW = [cos(psi), -sin(psi); sin(psi), cos(psi)];
    rotatedLeftWheel = (fW * leftWheelVertices')';
    rotatedRightWheel = (fW * rightWheelVertices')';
    rotatedRearLeftWheel = (rW * rearLeftWheelVertices')';
    rotatedRearRightWheel = (rW * rearRightWheelVertices')';
    
    translatedLW = rotatedLW + [x, y];
    translatedLeftWheel = rotatedLeftWheel + [x + cos(psi + pi/2) + cos(psi), y + sin(psi + pi/2) + sin(psi)];
    translatedRightWheel = rotatedRightWheel + [x + cos(psi - pi/2) + cos(psi), y + sin(psi - pi/2) + sin(psi)];
    translatedRearLeftWheel = rotatedRearLeftWheel + [x + cos(psi + pi/2) - cos(psi), y + sin(psi + pi/2) - sin(psi)];
    translatedRearRightWheel = rotatedRearRightWheel + [x + cos(psi - pi/2) - cos(psi), y + sin(psi - pi/2) - sin(psi)];
    
    set(leftWheelPatch, 'XData', translatedLeftWheel(:,1), 'YData', translatedLeftWheel(:,2));
    set(rightWheelPatch, 'XData', translatedRightWheel(:,1), 'YData', translatedRightWheel(:,2));
    set(rearLeftWheelPatch, 'XData', translatedRearLeftWheel(:,1), 'YData', translatedRearLeftWheel(:,2));
    set(rearRightWheelPatch, 'XData', translatedRearRightWheel(:,1), 'YData', translatedRearRightWheel(:,2));
    set(lwPatch, 'XData', translatedLW(:,1), 'YData', translatedLW(:,2));
    set(pathPlot, 'XData', vehiclePathX, 'YData', vehiclePathY);
    set(refPlot, 'XData', refPathX, 'YData', refPathY);
    
    xlim([x-20, x+20]);
    if x - 15 < xmin
        xmin = x-15;
    end
    if x + 15 > xmax
        xmax = x+15;
    end
    ylim([y-20, y+20]);
    if y - 15 < ymin
        ymin = y-15;
    end
    if y + 15 > ymax
        ymax = y+15;
    end
    subplot(3,6,4:6);
    xlim([time-10, time+2]);
    set(velocityPlot, 'XData', timeArray,'YData', velocityArray);
    set(throttlePlot, 'XData', timeArray,'YData', throttleArray);

    subplot(3,6,10:12);
    xlim([time-10, time+2]);
    set(deltaPlot, 'XData', timeArray, 'YData', deltaArray);

    subplot(3,6,16:18)
    xlim([time-10, time+2]);
    set(posErrorPlot, 'XData', timeArray, 'YData', errorArray);

    drawnow
end

== matlab function trippel_oppdatert_sim/Inputs/Loop reference 2 add 20 ==
  data: time_step input; array input; y output
function y = fcn(time_step, array)
    % index = mod(time_step, N_STEPS_REFERENCE) + 1;
    index = mod(time_step, 500) + 1; 
    y = array.data(index);
end

== matlab function trippel_oppdatert_sim/Subsystem3/MATLAB Function ==
  data: alpha input; Fc output; kappa input; Bc parameter; Cc parameter; Dc parameter; Ec parameter; alpha_peak parameter; kappa_peak parameter
function Fc = fcn(alpha, kappa, Bc, Cc, Dc, Ec, alpha_peak, kappa_peak)

alpha_norm = alpha/alpha_peak;
kappa_norm = kappa/kappa_peak;

S = sqrt(alpha_norm^2+kappa_norm^2);

alpha_mod = S * alpha_peak;

Fc = alpha_norm/S * Dc*sin(Cc*atan(Bc*alpha_mod-Ec*(Bc*alpha_mod-atan(Bc*alpha_mod))));

== matlab function trippel_oppdatert_sim/Subsystem2/MATLAB Function ==
  data: xd input; xdot output
function xdot = fcn(xd)

if xd == 0
    xdot = 0.001;
else
    xdot = xd;
end

== matlab function trippel_oppdatert_sim/Subsystem4/MATLAB Function ==
  data: xd input; xdot output
function xdot = fcn(xd)

if xd == 0
    xdot = 0.001;
else
    xdot = xd;
end

== matlab function trippel_oppdatert_sim/Inputs/Loop reference 2 ==
  data: time_step input; array input; y output
function y = fcn(time_step, array)
    % index = mod(time_step, N_STEPS_REFERENCE) + 1;
    index = mod(time_step, 500) + 1; 
    y = array.data(index);
end

== matlab function trippel_oppdatert_sim/Inputs/Loop reference ==
  data: time_step input; array input; y output
function y = fcn(time_step, array)
    % index = mod(time_step, N_STEPS_REFERENCE) + 1;
    index = mod(time_step, 500) + 1; 
    y = array.data(index);
end

== matlab function trippel_oppdatert_sim/MATLAB Function10 ==
  data: xdot input; v output; ydot input
function v = fcn(xdot, ydot)

v = sqrt(xdot^2+ydot^2);

== matlab function trippel_oppdatert_sim/Subsystem3/MATLAB Function11 ==
  data: Fl input; Fxf output; delta input
function Fxf = fcn(Fl, delta)

Fxf = Fl*cos(delta);

== matlab function trippel_oppdatert_sim/Subsystem4/MATLAB Function8 ==
  data: Fx output; Bl parameter; Cl parameter; Dl parameter; El parameter; kappa_peak parameter; alpha_peak parameter; kappa input; alpha input
function Fx = fcn(Bl, Cl, Dl, El, kappa_peak, alpha_peak, kappa, alpha)

alpha_norm = alpha/alpha_peak;
kappa_norm = kappa/kappa_peak;

S = sqrt(alpha_norm^2+kappa_norm^2);

kappa_mod = S * alpha_peak;

Fx = kappa_norm/S * Dl*sin(Cl*atan(Bl*kappa_mod-El*(Bl*kappa_mod-atan(Bl*kappa_mod))));
